simulink model "dspsrcnvf"  (Simulink 6.0)
settings: Solver=FixedStepDiscrete  SolverMode=SingleTasking  StartTime=0.0  StopTime=99.0  RelTol=1e-3  AbsTol=1e-6
libraries: dspsnks4 x4, dspsigops x4, dsparch4 x1, dspmlti3 x1, dspsrcs4 x1
settings Model: CovMetricSettings=d  Creator=edecosta  LastModifiedBy=sconahan  ExtModeTrigMode=oneshot  ExtModeArmWhenConnect=off  BufferReuse=off
settings DataIOCC: LimitDataPoints=off  SaveOutput=off  SaveTime=off  SignalLoggingName=sigsOut
settings OptimizationCC: BlockReduction=off  BooleanDataType=off  OptimizeBlockIOStorage=off  BufferReuse=off  LocalBlockOutputs=off  MultiInstanced=off  RollThreshold=2
settings FormatCC: IgnoreBidirectionalLines=off
settings DebuggingCC: IntegerOverflowMsg=none
settings HardwareCC: TargetUnknown=on
settings CodeAppCC: FileBanners=off  CustomSymbols=off
settings GRTTargetCC: TargetFcnLib=iso_c_tmw.mat  IsERTTarget=off

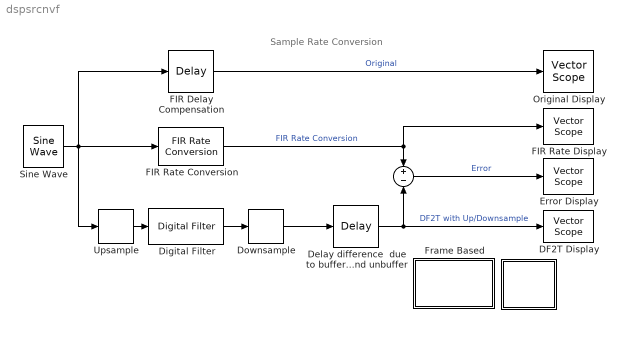
== system dspsrcnvf ==
  note: Sample Rate Conversion
  " " : Sum  Inputs=+-  SaturateOnIntegerOverflow=on  InputSameDT=on
  "  " : Subsystem
      mask Display: disp('Info')
  DF2T Display : dspsnks4/Vector Scope  ScopeProperties=on  Domain=Time  HorizSpan=10  DisplayProperties=off  AxisGrid=on  Memory=off  FrameNumber=off  AxisLegend=off  AxisZoom=on  OpenScopeAtSimStart=on  OpenScopeImmediately=off  FigPos=[650 381 544 176]  AxisProperties=off  XUnits=Hertz  XRange=[0...Fs/2]  InheritXIncr=on  XIncr=1  XLabel=Samples  YUnits=dB  YLabel=Amplitude  LineProperties=off  LineColors=blue
      settings: YMin=-1.1  YMax=1.1
  Delay difference  due to buffer  and unbuffer : dspsigops/Delay  dly_unit=Samples  delay=32  ic_detail=on  dif_ic_for_ch=off  dif_ic_for_dly=off  ic=0  reset_popup=None
  Digital Filter : dsparch4/Digital Filter  TypePopup=FIR (all zeros)  IIRFiltStruct=Direct form II transposed  AllPoleFiltStruct=Direct form  FIRFiltStruct=Direct form  CoeffSource=Specify via dialog  NumCoeffs=fir1(63,1/8)*8  DenCoeffs=[1 0.1]  BiQuadCoeffs=[1 0.3 0.4 1 0.1 0.2]  LatticeCoeffs=[0.2 0.4]  denIgnore=on  FiltPerSampPopup=One filter per frame  IC=0  ICnum=0  ICden=0  roundingMode=Floor  overflowMode=off
  Downsample : dspsigops/Downsample  N=5  phase=0  ic=0  smode=Allow multirate  fmode=Maintain input frame rate
  Error Display : dspsnks4/Vector Scope  ScopeProperties=on  Domain=Time  HorizSpan=10  DisplayProperties=off  AxisGrid=on  Memory=off  FrameNumber=off  AxisLegend=off  AxisZoom=on  OpenScopeAtSimStart=on  OpenScopeImmediately=off  FigPos=[77 382 560 176]  AxisProperties=off  XUnits=Hertz  XRange=[0...Fs/2]  InheritXIncr=on  XIncr=1  XLabel=Samples  YUnits=dB  YLabel=Amplitude  LineProperties=off  LineColors=red
      settings: YMin=-0.01  YMax=0.01
  FIR Delay Compensation : dspsigops/Delay  dly_unit=Samples  delay="[5 + round(5/8 * 63/2 -1)  ]"  ic_detail=on  dif_ic_for_ch=off  dif_ic_for_dly=off  ic=0  reset_popup=None
  FIR Rate Conversion : dspmlti3/FIR Rate Conversion  L=8  h=fir1(63,1/8)*8  M=5  roundingMode=Floor  overflowMode=off
  "FIR Rate Display " : dspsnks4/Vector Scope  ScopeProperties=on  Domain=Time  HorizSpan=10  DisplayProperties=off  AxisGrid=on  Memory=off  FrameNumber=off  AxisLegend=off  AxisZoom=on  OpenScopeAtSimStart=on  OpenScopeImmediately=off  FigPos=[651 583 545 179]  AxisProperties=off  XUnits=Hertz  XRange=[0...Fs/2]  InheritXIncr=on  XIncr=1  XLabel=Samples  YUnits=dB  YLabel=Amplitude  LineProperties=off
      settings: YMin=-1.1  YMax=1.1
  Frame Based : Subsystem
      settings: OpenFcn=dspsrcnv;
      mask Display: disp('Sample-based\nVersion')
  Original Display : dspsnks4/Vector Scope  ScopeProperties=on  Domain=Time  HorizSpan=10  DisplayProperties=off  AxisGrid=on  Memory=off  FrameNumber=off  AxisLegend=off  AxisZoom=on  OpenScopeAtSimStart=on  OpenScopeImmediately=off  FigPos=[649 790 545 178]  AxisProperties=off  XUnits=Hertz  XRange=[0...Fs/2]  InheritXIncr=on  XIncr=1  XLabel=Samples  YUnits=dB  YLabel=Amplitude  LineProperties=off  LineColors=green
      settings: YMin=-1.1  YMax=1.1
  Sine Wave : dspsrcs4/Sine Wave  Amplitude=1  Frequency=0.1  Phase=0  SampleMode=Discrete  OutComplex=Real  CompMethod=Trigonometric fcn  TableSize=Speed  SampleTime=1  SamplesPerFrame=10  dataType=double  wordLen=16  udDataType=sfix(16)  fracBitsMode=Best precision  numFracBits=14  ResetState=Restart at time zero
  Upsample : dspsigops/Upsample  N=8  phase=0  ic=0  mode=Maintain input frame rate
  wires:
  Sine Wave/1 -> Upsample/1, FIR Rate Conversion/1, FIR Delay Compensation/1
  Upsample/1 -> Digital Filter/1
  Digital Filter/1 -> Downsample/1
  FIR Rate Conversion/1 -> "FIR Rate Display "/1, " "/1  "FIR Rate Conversion"
  FIR Delay Compensation/1 -> Original Display/1  "Original"
  Downsample/1 -> Delay difference  due to buffer  and unbuffer/1
  Delay difference  due to buffer  and unbuffer/1 -> " "/2, DF2T Display/1  "DF2T with Up/Downsample"
  " "/1 -> Error Display/1  "Error"

== system dspsrcnvf/   ==
  note: Digital Sample Rate Conversion:
      |         Frame-Based Implementation
  note: This system demonstrates the equivalence between the "FIR
      | Rate Conversion"  block and the straightforward but far less
      | efficient system consisting of separate upsampling, FIR filtering,
      | and downsampling blocks.  Note that there is a delay
      | between the input signal and the rate-conversion result.
      |
      | Efficiency is gained by employing a polyphase implementation
      | for up- and down-sampling.  This technique effectively eliminates
      | all multiplication by zeros (during the interpolation process) and
      | computation of discarded outputs (during the decimation process).
      |
      | The rate conversion must be chosen to be a ratio of relatively
      | prime integers, such as the 8/5 used in the example.  An arbitrary
      | integer ratio may be easily converted to a relatively prime ratio
      | by dividing by the GCD (greatest common divisor).
  note: The filter is used to bandlimit the signal to 1/max(M,L), where M and L
      | are the downsampling and upsampling factors, respectively.
      | Filter order should be sufficiently high so as to yield satisfactory
      | reduction of aliasing and imaging artifacts.
      |
      | Compare the execution speed of this demo vs. that of
      | the sample-based implementation.

== system dspsrcnvf/Frame Based ==
